simulink library "RspLib"  (R2018b)
settings: Solver=VariableStepAuto  StartTime=0.0  StopTime=10.0  RelTol=1e-3
undefined symbols (not defined in the file or in its folder): HMIRsp1, PassRsp1, RclRspStat1
libraries: $bdroot x22
settings Model: Creator=sn2xws  LastModifiedBy=sn2xws

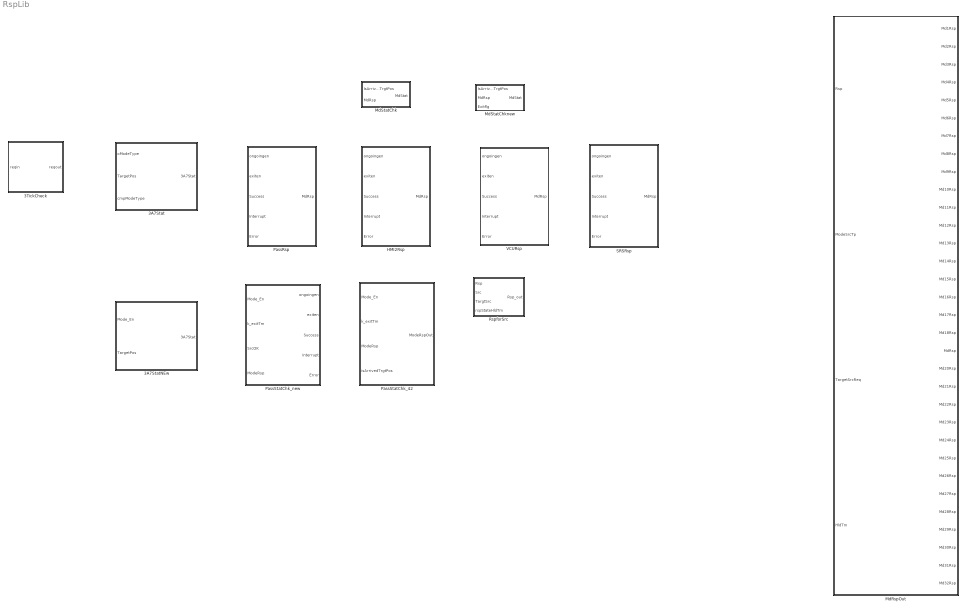
== system RspLib ==
  3A7Stat : Subsystem
  3A7StatNEw : Subsystem
  3TickCheck : Subsystem
  HMI2Rsp : Subsystem
  MdRspOut : Subsystem
  MdStatChk : Subsystem
  MdStatChknew : Subsystem
  PassRsp : Subsystem
  PassStatChk_42 : Stateflow chart  TreatAsAtomicUnit=on
  PassStatChk_new : Stateflow chart  TreatAsAtomicUnit=on
  RspforSrc : Subsystem
  SRSRsp : Subsystem
  VCURsp : Subsystem

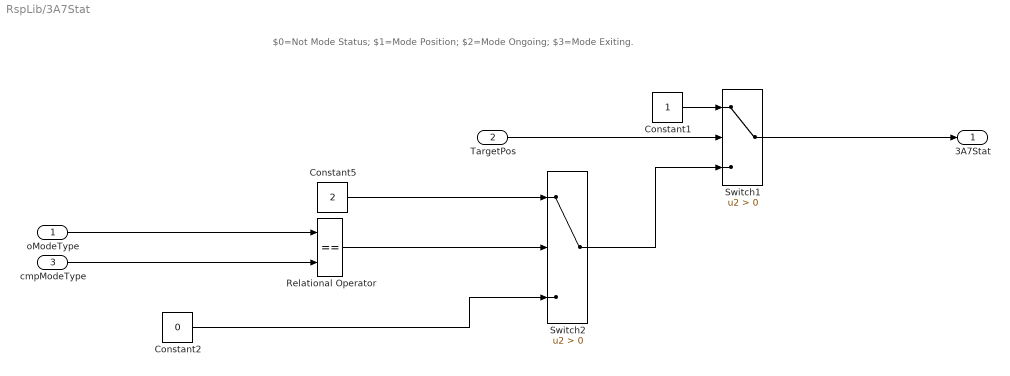
== system RspLib/3A7Stat ==
  note: $0=Not Mode Status; $1=Mode Position; $2=Mode Ongoing; $3=Mode Exiting.
  oModeType : Inport
  TargetPos : Inport  Port=2
  cmpModeType : Inport  Port=3
  Constant1 : Constant  OutDataTypeStr=uint8
  Constant2 : Constant  Value=0  OutDataTypeStr=uint8
  Constant5 : Constant  Value=2  OutDataTypeStr=uint8
  Relational Operator : RelationalOperator  Operator===  OutDataTypeStr=boolean  RndMeth=Simplest
  Switch1 : Switch  Criteria=u2 > Threshold
  Switch2 : Switch  Criteria=u2 > Threshold
  3A7Stat : Outport
  wires:
  Constant5/1 -> Switch2/1
  cmpModeType/1 -> Relational Operator/2
  TargetPos/1 -> Switch1/2
  Constant1/1 -> Switch1/1
  Relational Operator/1 -> Switch2/2
  oModeType/1 -> Relational Operator/1
  Switch1/1 -> 3A7Stat/1
  Constant2/1 -> Switch2/3
  Switch2/1 -> Switch1/3

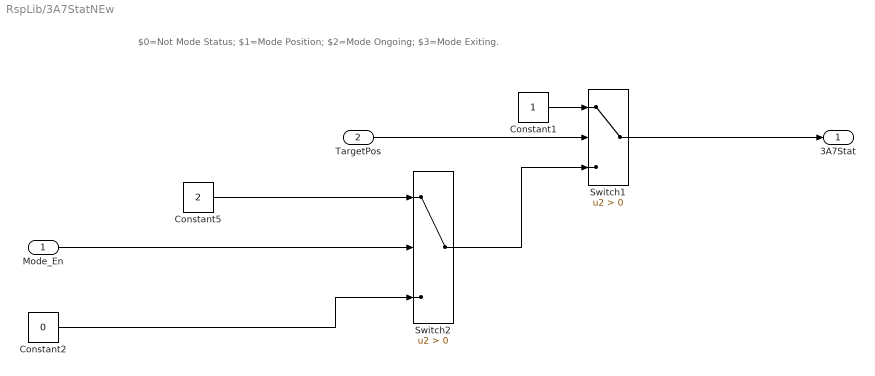
== system RspLib/3A7StatNEw ==
  note: $0=Not Mode Status; $1=Mode Position; $2=Mode Ongoing; $3=Mode Exiting.
  Mode_En : Inport
  TargetPos : Inport  Port=2
  Constant1 : Constant  OutDataTypeStr=uint8
  Constant2 : Constant  Value=0  OutDataTypeStr=uint8
  Constant5 : Constant  Value=2  OutDataTypeStr=uint8
  Switch1 : Switch  Criteria=u2 > Threshold
  Switch2 : Switch  Criteria=u2 > Threshold
  3A7Stat : Outport
  wires:
  Switch2/1 -> Switch1/3
  Constant2/1 -> Switch2/3
  Switch1/1 -> 3A7Stat/1
  Constant1/1 -> Switch1/1
  TargetPos/1 -> Switch1/2
  Constant5/1 -> Switch2/1
  Mode_En/1 -> Switch2/2

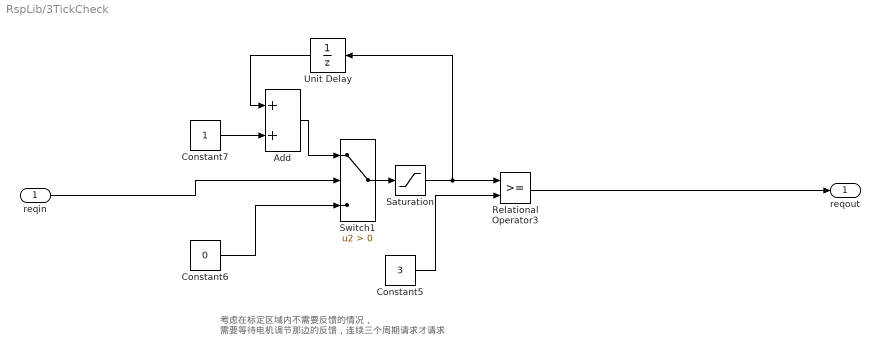
== system RspLib/3TickCheck ==
  note: 考虑在标定区域内不需要反馈的情况，
      | 需要等待电机调节那边的反馈，连续三个周期请求才请求
  reqin : Inport
  Add : Sum
  Constant5 : Constant  Value=3  OutDataTypeStr=uint8
  Constant6 : Constant  Value=0  OutDataTypeStr=uint8
  Constant7 : Constant  OutDataTypeStr=uint8
  Relational Operator3 : RelationalOperator  OutDataTypeStr=boolean  RndMeth=Simplest
  Saturation : Saturate  UpperLimit=3  LowerLimit=0  OutDataTypeStr=uint8
  Switch1 : Switch  Criteria=u2 > Threshold
  Unit Delay : UnitDelay  SampleTime=-1
  reqout : Outport
  wires:
  Unit Delay/1 -> Add/1
  Constant6/1 -> Switch1/3
  Constant5/1 -> Relational Operator3/2
  Constant7/1 -> Add/2
  Saturation/1 -> Unit Delay/1, Relational Operator3/1
  Add/1 -> Switch1/1
  Switch1/1 -> Saturation/1
  reqin/1 -> Switch1/2
  Relational Operator3/1 -> reqout/1

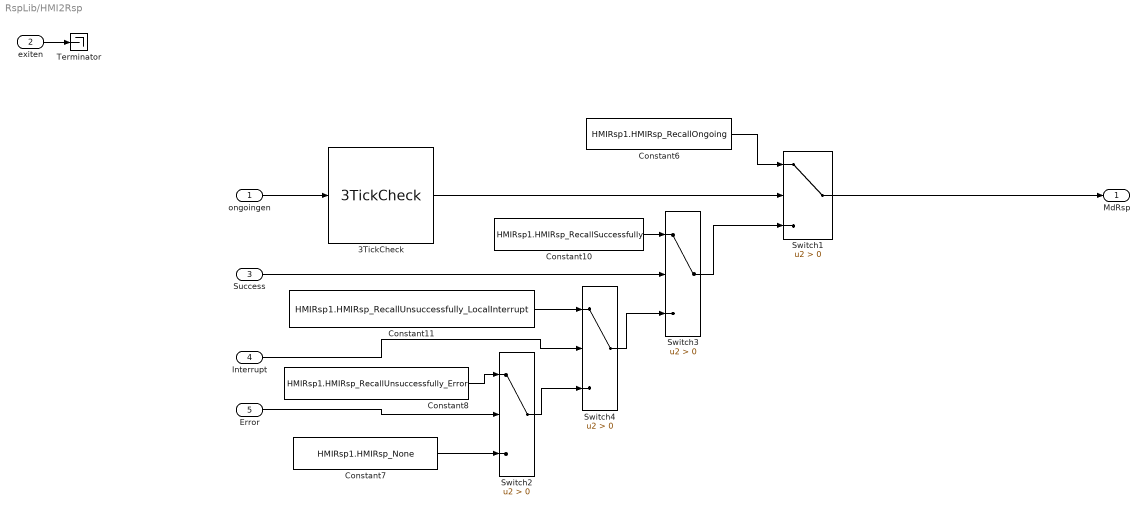
== system RspLib/HMI2Rsp ==
  ongoingen : Inport
  exiten : Inport  Port=2
  Success : Inport  Port=3
  Interrupt : Inport  Port=4
  Error : Inport  Port=5
  3TickCheck : $bdroot/3TickCheck  SystemSampleTime=-1
  Constant10 : Constant  Value=HMIRsp1.HMIRsp_RecallSuccessfully  OutDataTypeStr=Enum:HMIRsp1  SampleTime=-1
  Constant11 : Constant  Value=HMIRsp1.HMIRsp_RecallUnsuccessfully_LocalInterrupt  OutDataTypeStr=Enum:HMIRsp1  SampleTime=-1
  Constant6 : Constant  Value=HMIRsp1.HMIRsp_RecallOngoing  OutDataTypeStr=Enum:HMIRsp1  SampleTime=-1
  Constant7 : Constant  Value=HMIRsp1.HMIRsp_None  OutDataTypeStr=Enum:HMIRsp1  SampleTime=-1
  Constant8 : Constant  Value=HMIRsp1.HMIRsp_RecallUnsuccessfully_Error  OutDataTypeStr=Enum:HMIRsp1  SampleTime=-1
  Switch{1..4} (4 alike) : Switch  Criteria=u2 > Threshold
  Terminator : Terminator
  MdRsp : Outport  VectorParamsAs1DForOutWhenUnconnected=on
  wires:
  Constant10/1 -> Switch3/1
  Switch3/1 -> Switch1/3
  Switch1/1 -> MdRsp/1
  Constant6/1 -> Switch1/1
  Success/1 -> Switch3/2
  Switch2/1 -> Switch4/3
  Constant8/1 -> Switch2/1
  Constant11/1 -> Switch4/1
  Constant7/1 -> Switch2/3
  Switch4/1 -> Switch3/3
  ongoingen/1 -> 3TickCheck/1
  Interrupt/1 -> Switch4/2
  Error/1 -> Switch2/2
  exiten/1 -> Terminator/1
  3TickCheck/1 -> Switch1/2

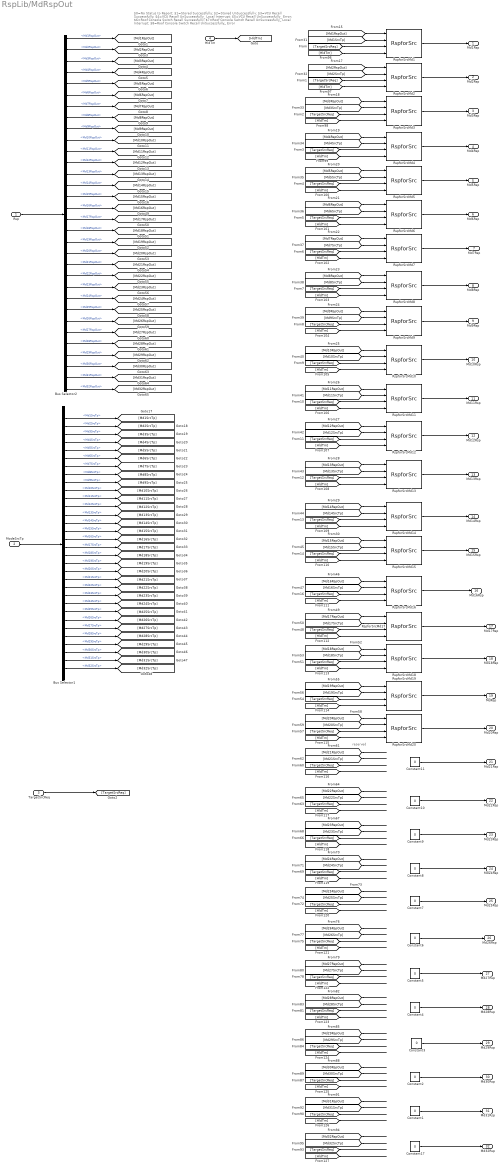
== system RspLib/MdRspOut ==
  note: $0=No Status to Report; $1=Stored Successfully; $2=Stored UnSuccessfully; $3=VCU Recall Successfully; $4=VCU Recall UnSuccessfully_ Local Interrupt; $5=VCU Recall UnSuccessfully_ Error; $6=Roof Console Switch Recall Successfully; $7=Roof Console Switch Recall UnSuccessfully_ Local Interrupt; $8=Roof Console Switch Recall UnSuccessfully_ Error
  note: reserved
  Rsp : Inport
  ModeSrcTp : Inport  Port=2
  TargetSrcReq : Inport  Port=3
  HldTm : Inport  Port=4
  Bus Selector1 : BusSelector  OutputSignals=Md1SrcTp,Md2SrcTp,Md3SrcTp,Md4SrcTp,Md5SrcTp,Md6SrcTp,Md7SrcTp,Md8SrcTp,Md9SrcTp,Md10SrcTp,Md11SrcTp,Md12SrcTp,Md13SrcTp,Md14SrcTp,Md15SrcTp,Md16SrcTp,Md17SrcTp,Md18SrcTp,Md19SrcTp,Md20SrcTp,Md21SrcTp,Md22SrcTp,Md23SrcTp,Md24SrcTp,Md25SrcTp,Md26SrcTp,Md27SrcTp,Md28SrcTp,Md29SrcTp,Md30SrcTp,Md31SrcTp,Md32SrcTp
  Bus Selector2 : BusSelector  OutputSignals=Md1RspOut,Md2RspOut,Md3RspOut,Md4RspOut,Md5RspOut,Md6RspOut,Md7RspOut,Md8RspOut,Md9RspOut,Md10RspOut,Md11RspOut,Md12RspOut,Md13RspOut,Md14RspOut,Md15RspOut,Md16RspOut,Md17RspOut,Md18RspOut,Md19RspOut,Md20RspOut,Md21RspOut,Md22RspOut,Md23RspOut,Md24RspOut,Md25RspOut,Md26RspOut,Md27RspOut,Md28RspOut,Md29RspOut,Md30RspOut,Md31RspOut,Md32RspOut
  Constant{1..11,17} (12 alike) : Constant  Value=0  OutDataTypeStr=uint8
  RspforSrcMd{1..20} (20 alike) : $bdroot/RspforSrc  SystemSampleTime=-1
  Md1Rsp : Outport  VectorParamsAs1DForOutWhenUnconnected=on
  Md2Rsp : Outport  Port=2  VectorParamsAs1DForOutWhenUnconnected=on
  Md3Rsp : Outport  Port=3  VectorParamsAs1DForOutWhenUnconnected=on
  Md4Rsp : Outport  Port=4  VectorParamsAs1DForOutWhenUnconnected=on
  Md5Rsp : Outport  Port=5  VectorParamsAs1DForOutWhenUnconnected=on
  Md6Rsp : Outport  Port=6  VectorParamsAs1DForOutWhenUnconnected=on
  Md7Rsp : Outport  Port=7  VectorParamsAs1DForOutWhenUnconnected=on
  Md8Rsp : Outport  Port=8  VectorParamsAs1DForOutWhenUnconnected=on
  Md9Rsp : Outport  Port=9  VectorParamsAs1DForOutWhenUnconnected=on
  Md10Rsp : Outport  Port=10  VectorParamsAs1DForOutWhenUnconnected=on
  Md11Rsp : Outport  Port=11  VectorParamsAs1DForOutWhenUnconnected=on
  Md12Rsp : Outport  Port=12  VectorParamsAs1DForOutWhenUnconnected=on
  Md13Rsp : Outport  Port=13  VectorParamsAs1DForOutWhenUnconnected=on
  Md14Rsp : Outport  Port=14  VectorParamsAs1DForOutWhenUnconnected=on
  Md15Rsp : Outport  Port=15  VectorParamsAs1DForOutWhenUnconnected=on
  Md16Rsp : Outport  Port=16  VectorParamsAs1DForOutWhenUnconnected=on
  Md17Rsp : Outport  Port=17  VectorParamsAs1DForOutWhenUnconnected=on
  Md18Rsp : Outport  Port=18  VectorParamsAs1DForOutWhenUnconnected=on
  MdRsp : Outport  Port=19  VectorParamsAs1DForOutWhenUnconnected=on
  Md20Rsp : Outport  Port=20  VectorParamsAs1DForOutWhenUnconnected=on
  Md21Rsp : Outport  Port=21  VectorParamsAs1DForOutWhenUnconnected=on
  Md22Rsp : Outport  Port=22  VectorParamsAs1DForOutWhenUnconnected=on
  Md23Rsp : Outport  Port=23  VectorParamsAs1DForOutWhenUnconnected=on
  Md24Rsp : Outport  Port=24  VectorParamsAs1DForOutWhenUnconnected=on
  Md25Rsp : Outport  Port=25  VectorParamsAs1DForOutWhenUnconnected=on
  Md26Rsp : Outport  Port=26  VectorParamsAs1DForOutWhenUnconnected=on
  Md27Rsp : Outport  Port=27  VectorParamsAs1DForOutWhenUnconnected=on
  Md28Rsp : Outport  Port=28  VectorParamsAs1DForOutWhenUnconnected=on
  Md29Rsp : Outport  Port=29  VectorParamsAs1DForOutWhenUnconnected=on
  Md30Rsp : Outport  Port=30  VectorParamsAs1DForOutWhenUnconnected=on
  Md31Rsp : Outport  Port=31  VectorParamsAs1DForOutWhenUnconnected=on
  Md32Rsp : Outport  Port=32  VectorParamsAs1DForOutWhenUnconnected=on
  wires:
  [TargetSrcReq] -> ?
  [Md32RspOut] -> ?
  [Md32SrcTp] -> ?
  [Md31SrcTp] -> ?
  [Md31RspOut] -> ?
  [TargetSrcReq] -> ?
  [TargetSrcReq] -> ?
  [Md30RspOut] -> ?
  [Md30SrcTp] -> ?
  [Md29SrcTp] -> ?
  [Md29RspOut] -> ?
  [TargetSrcReq] -> ?
  [TargetSrcReq] -> ?
  [Md28RspOut] -> ?
  [Md28SrcTp] -> ?
  [Md27SrcTp] -> ?
  [Md27RspOut] -> ?
  [TargetSrcReq] -> ?
  [TargetSrcReq] -> ?
  [Md26RspOut] -> ?
  [Md26SrcTp] -> ?
  [Md25SrcTp] -> ?
  [Md25RspOut] -> ?
  [TargetSrcReq] -> ?
  [TargetSrcReq] -> ?
  [Md24RspOut] -> ?
  [Md24SrcTp] -> ?
  [Md23SrcTp] -> ?
  [Md23RspOut] -> ?
  [TargetSrcReq] -> ?
  [TargetSrcReq] -> ?
  [Md22RspOut] -> ?
  [Md22SrcTp] -> ?
  [Md21SrcTp] -> ?
  [Md21RspOut] -> ?
  [TargetSrcReq] -> ?
  [TargetSrcReq] -> RspforSrcMd20/3
  [Md20RspOut] -> RspforSrcMd20/1
  [Md20SrcTp] -> RspforSrcMd20/2
  [Md19SrcTp] -> RspforSrcMd19/2
  [Md19RspOut] -> RspforSrcMd19/1
  [TargetSrcReq] -> RspforSrcMd19/3
  [TargetSrcReq] -> RspforSrcMd18/3
  [Md18RspOut] -> RspforSrcMd18/1
  [Md18SrcTp] -> RspforSrcMd18/2
  Bus Selector2/32 -> [Md32RspOut]  "<Md32RspOut>"
  Bus Selector2/31 -> [Md31RspOut]  "<Md31RspOut>"
  Bus Selector2/30 -> [Md30RspOut]  "<Md30RspOut>"
  Bus Selector2/29 -> [Md29RspOut]  "<Md29RspOut>"
  Bus Selector2/28 -> [Md28RspOut]  "<Md28RspOut>"
  Bus Selector2/27 -> [Md27RspOut]  "<Md27RspOut>"
  Bus Selector2/26 -> [Md26RspOut]  "<Md26RspOut>"
  Bus Selector2/25 -> [Md25RspOut]  "<Md25RspOut>"
  Bus Selector2/24 -> [Md24RspOut]  "<Md24RspOut>"
  Bus Selector2/23 -> [Md23RspOut]  "<Md23RspOut>"
  Bus Selector2/22 -> [Md22RspOut]  "<Md22RspOut>"
  Bus Selector2/21 -> [Md21RspOut]  "<Md21RspOut>"
  Bus Selector2/20 -> [Md20RspOut]  "<Md20RspOut>"
  Bus Selector2/19 -> [Md19RspOut]  "<Md19RspOut>"
  Bus Selector2/18 -> [Md18RspOut]  "<Md18RspOut>"
  Bus Selector2/17 -> [Md17RspOut]  "<Md17RspOut>"
  Bus Selector2/16 -> [Md16RspOut]  "<Md16RspOut>"
  [Md17SrcTp] -> RspforSrcMd17/2
  [Md17RspOut] -> RspforSrcMd17/1
  [TargetSrcReq] -> RspforSrcMd17/3
  [TargetSrcReq] -> RspforSrcMd16/3
  [Md16RspOut] -> RspforSrcMd16/1
  [Md16SrcTp] -> RspforSrcMd16/2
  Bus Selector1/32 -> [Md32SrcTp]  "<Md32SrcTp>"
  Bus Selector1/31 -> [Md31SrcTp]  "<Md31SrcTp>"
  Bus Selector1/30 -> [Md30SrcTp]  "<Md30SrcTp>"
  Bus Selector1/29 -> [Md29SrcTp]  "<Md29SrcTp>"
  Bus Selector1/28 -> [Md28SrcTp]  "<Md28SrcTp>"
  Bus Selector1/27 -> [Md27SrcTp]  "<Md27SrcTp>"
  Bus Selector1/26 -> [Md26SrcTp]  "<Md26SrcTp>"
  Bus Selector1/25 -> [Md25SrcTp]  "<Md25SrcTp>"
  Bus Selector1/24 -> [Md24SrcTp]  "<Md24SrcTp>"
  Bus Selector1/23 -> [Md23SrcTp]  "<Md23SrcTp>"
  Bus Selector1/22 -> [Md22SrcTp]  "<Md22SrcTp>"
  Bus Selector1/21 -> [Md21SrcTp]  "<Md21SrcTp>"
  Bus Selector1/20 -> [Md20SrcTp]  "<Md20SrcTp>"
  Bus Selector1/19 -> [Md19SrcTp]  "<Md19SrcTp>"
  Bus Selector1/18 -> [Md18SrcTp]  "<Md18SrcTp>"
  Bus Selector1/17 -> [Md17SrcTp]  "<Md17SrcTp>"
  Bus Selector1/16 -> [Md16SrcTp]  "<Md16SrcTp>"
  [Md14SrcTp] -> RspforSrcMd14/2
  [Md13SrcTp] -> RspforSrcMd13/2
  [Md15SrcTp] -> RspforSrcMd15/2
  [Md12SrcTp] -> RspforSrcMd12/2
  [Md11SrcTp] -> RspforSrcMd11/2
  [Md10SrcTp] -> RspforSrcMd10/2
  [Md9SrcTp] -> RspforSrcMd9/2
  [Md8SrcTp] -> RspforSrcMd8/2
  [Md7SrcTp] -> RspforSrcMd7/2
  [Md6SrcTp] -> RspforSrcMd6/2
  [Md5SrcTp] -> RspforSrcMd5/2
  [Md4SrcTp] -> RspforSrcMd4/2
  [Md3SrcTp] -> RspforSrcMd3/2
  [Md2SrcTp] -> RspforSrcMd2/2
  Bus Selector1/15 -> [Md15SrcTp]  "<Md15SrcTp>"
  Bus Selector1/14 -> [Md14SrcTp]  "<Md14SrcTp>"
  Bus Selector1/13 -> [Md13SrcTp]  "<Md13SrcTp>"
  Bus Selector1/12 -> [Md12SrcTp]  "<Md12SrcTp>"
  Bus Selector1/11 -> [Md11SrcTp]  "<Md11SrcTp>"
  Bus Selector1/10 -> [Md10SrcTp]  "<Md10SrcTp>"
  Bus Selector1/9 -> [Md9SrcTp]  "<Md9SrcTp>"
  Bus Selector1/8 -> [Md8SrcTp]  "<Md8SrcTp>"
  Bus Selector1/7 -> [Md7SrcTp]  "<Md7SrcTp>"
  Bus Selector1/6 -> [Md6SrcTp]  "<Md6SrcTp>"
  Bus Selector1/5 -> [Md5SrcTp]  "<Md5SrcTp>"
  Bus Selector1/4 -> [Md4SrcTp]  "<Md4SrcTp>"
  Bus Selector1/3 -> [Md3SrcTp]  "<Md3SrcTp>"
  Bus Selector1/2 -> [Md2SrcTp]  "<Md2SrcTp>"
  Bus Selector1/1 -> [Md1SrcTp]  "<Md1SrcTp>"
  Constant7/1 -> Md25Rsp/1
  [Md15RspOut] -> RspforSrcMd15/1
  [Md14RspOut] -> RspforSrcMd14/1
  [Md13RspOut] -> RspforSrcMd13/1
  [Md12RspOut] -> RspforSrcMd12/1
  [Md11RspOut] -> RspforSrcMd11/1
  [Md10RspOut] -> RspforSrcMd10/1
  [Md9RspOut] -> RspforSrcMd9/1
  [Md8RspOut] -> RspforSrcMd8/1
  [Md7RspOut] -> RspforSrcMd7/1
  [Md6RspOut] -> RspforSrcMd6/1
  [Md5RspOut] -> RspforSrcMd5/1
  [Md4RspOut] -> RspforSrcMd4/1
  [Md3RspOut] -> RspforSrcMd3/1
  [Md2RspOut] -> RspforSrcMd2/1
  RspforSrcMd15/1 -> Md15Rsp/1
  RspforSrcMd14/1 -> Md14Rsp/1
  RspforSrcMd13/1 -> Md13Rsp/1
  RspforSrcMd12/1 -> Md12Rsp/1
  RspforSrcMd11/1 -> Md11Rsp/1
  RspforSrcMd10/1 -> Md10Rsp/1
  RspforSrcMd9/1 -> Md9Rsp/1
  RspforSrcMd8/1 -> Md8Rsp/1
  RspforSrcMd7/1 -> Md7Rsp/1
  RspforSrcMd6/1 -> Md6Rsp/1
  RspforSrcMd5/1 -> Md5Rsp/1
  RspforSrcMd4/1 -> Md4Rsp/1
  RspforSrcMd3/1 -> Md3Rsp/1
  RspforSrcMd2/1 -> Md2Rsp/1
  RspforSrcMd1/1 -> Md1Rsp/1
  [TargetSrcReq] -> RspforSrcMd1/3
  [Md1SrcTp] -> RspforSrcMd1/2
  [Md1RspOut] -> RspforSrcMd1/1
  [TargetSrcReq] -> RspforSrcMd15/3
  [TargetSrcReq] -> RspforSrcMd14/3
  [TargetSrcReq] -> RspforSrcMd13/3
  [TargetSrcReq] -> RspforSrcMd12/3
  [TargetSrcReq] -> RspforSrcMd11/3
  RspforSrcMd17/1 -> Md17Rsp/1
  RspforSrcMd18/1 -> Md18Rsp/1
  RspforSrcMd19/1 -> MdRsp/1
  RspforSrcMd20/1 -> Md20Rsp/1
  Constant11/1 -> Md21Rsp/1
  Constant10/1 -> Md22Rsp/1
  Constant9/1 -> Md23Rsp/1
  Constant8/1 -> Md24Rsp/1
  Constant6/1 -> Md26Rsp/1
  [TargetSrcReq] -> RspforSrcMd10/3
  [TargetSrcReq] -> RspforSrcMd9/3
  [TargetSrcReq] -> RspforSrcMd8/3
  [TargetSrcReq] -> RspforSrcMd7/3
  [TargetSrcReq] -> RspforSrcMd6/3
  [TargetSrcReq] -> RspforSrcMd5/3
  [TargetSrcReq] -> RspforSrcMd4/3
  [TargetSrcReq] -> RspforSrcMd3/3
  [TargetSrcReq] -> RspforSrcMd2/3
  Bus Selector2/15 -> [Md15RspOut]  "<Md15RspOut>"
  Bus Selector2/14 -> [Md14RspOut]  "<Md14RspOut>"
  Bus Selector2/13 -> [Md13RspOut]  "<Md13RspOut>"
  Bus Selector2/12 -> [Md12RspOut]  "<Md12RspOut>"
  Bus Selector2/11 -> [Md11RspOut]  "<Md11RspOut>"
  Bus Selector2/10 -> [Md10RspOut]  "<Md10RspOut>"
  Bus Selector2/9 -> [Md9RspOut]  "<Md9RspOut>"
  Bus Selector2/8 -> [Md8RspOut]  "<Md8RspOut>"
  Bus Selector2/7 -> [Md7RspOut]  "<Md7RspOut>"
  Bus Selector2/6 -> [Md6RspOut]  "<Md6RspOut>"
  Bus Selector2/5 -> [Md5RspOut]  "<Md5RspOut>"
  Bus Selector2/4 -> [Md4RspOut]  "<Md4RspOut>"
  Bus Selector2/3 -> [Md3RspOut]  "<Md3RspOut>"
  Bus Selector2/2 -> [Md2RspOut]  "<Md2RspOut>"
  Bus Selector2/1 -> [Md1RspOut]  "<Md1RspOut>"
  TargetSrcReq/1 -> [TargetSrcReq]
  ModeSrcTp/1 -> Bus Selector1/1
  Constant5/1 -> Md27Rsp/1
  Constant4/1 -> Md28Rsp/1
  Constant3/1 -> Md29Rsp/1
  Constant2/1 -> Md30Rsp/1
  Constant1/1 -> Md31Rsp/1
  Constant17/1 -> Md32Rsp/1
  Rsp/1 -> Bus Selector2/1
  [HldTm] -> RspforSrcMd1/4
  [HldTm] -> RspforSrcMd2/4
  [HldTm] -> RspforSrcMd3/4
  [HldTm] -> RspforSrcMd4/4
  [HldTm] -> RspforSrcMd5/4
  [HldTm] -> RspforSrcMd6/4
  [HldTm] -> RspforSrcMd7/4
  [HldTm] -> RspforSrcMd8/4
  [HldTm] -> RspforSrcMd9/4
  [HldTm] -> RspforSrcMd10/4
  [HldTm] -> RspforSrcMd11/4
  [HldTm] -> RspforSrcMd12/4
  [HldTm] -> RspforSrcMd13/4
  [HldTm] -> RspforSrcMd14/4
  [HldTm] -> RspforSrcMd15/4
  [HldTm] -> RspforSrcMd16/4
  [HldTm] -> RspforSrcMd17/4
  [HldTm] -> RspforSrcMd18/4
  [HldTm] -> RspforSrcMd19/4
  [HldTm] -> RspforSrcMd20/4
  [HldTm] -> ?
  [HldTm] -> ?
  [HldTm] -> ?
  [HldTm] -> ?
  [HldTm] -> ?
  [HldTm] -> ?
  [HldTm] -> ?
  [HldTm] -> ?
  [HldTm] -> ?
  [HldTm] -> ?
  [HldTm] -> ?
  [HldTm] -> ?
  HldTm/1 -> [HldTm]
  RspforSrcMd16/1 -> Md16Rsp/1

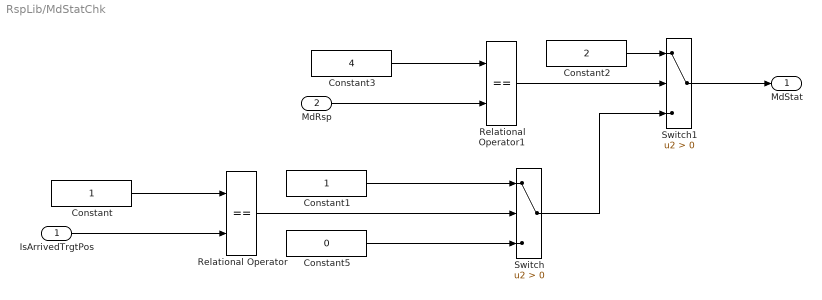
== system RspLib/MdStatChk ==
  IsArrivedTrgtPos : Inport
  MdRsp : Inport  Port=2
  Constant : Constant  OutDataTypeStr=boolean
  Constant1 : Constant  OutDataTypeStr=uint8
  Constant2 : Constant  Value=2  OutDataTypeStr=uint8
  Constant3 : Constant  Value=4  OutDataTypeStr=uint8
  Constant5 : Constant  Value=0  OutDataTypeStr=uint8
  Relational Operator : RelationalOperator  Operator===  OutDataTypeStr=boolean  RndMeth=Simplest
  Relational Operator1 : RelationalOperator  Operator===  OutDataTypeStr=boolean  RndMeth=Simplest
  Switch : Switch  Criteria=u2 > Threshold
  Switch1 : Switch  Criteria=u2 > Threshold
  MdStat : Outport
  wires:
  Constant3/1 -> Relational Operator1/1
  MdRsp/1 -> Relational Operator1/2
  Constant2/1 -> Switch1/1
  Relational Operator1/1 -> Switch1/2
  Constant1/1 -> Switch/1
  Constant/1 -> Relational Operator/1
  IsArrivedTrgtPos/1 -> Relational Operator/2
  Relational Operator/1 -> Switch/2
  Constant5/1 -> Switch/3
  Switch/1 -> Switch1/3
  Switch1/1 -> MdStat/1

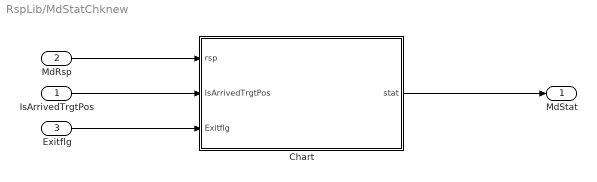
== system RspLib/MdStatChknew ==
  IsArrivedTrgtPos : Inport
  MdRsp : Inport  Port=2
  Exitflg : Inport  Port=3
  Chart : Stateflow chart  TreatAsAtomicUnit=on
  MdStat : Outport
  wires:
  MdRsp/1 -> Chart/1(rsp)
  Exitflg/1 -> Chart/3(Exitflg)
  IsArrivedTrgtPos/1 -> Chart/2(IsArrivedTrgtPos)
  Chart/1(stat) -> MdStat/1

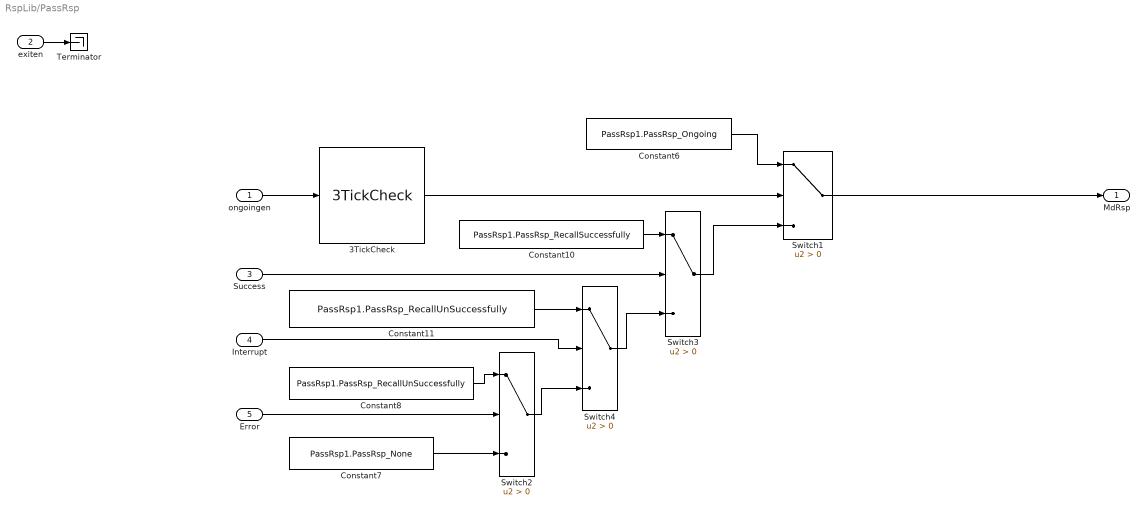
== system RspLib/PassRsp ==
  ongoingen : Inport
  exiten : Inport  Port=2
  Success : Inport  Port=3
  Interrupt : Inport  Port=4
  Error : Inport  Port=5
  3TickCheck : $bdroot/3TickCheck  SystemSampleTime=-1
  Constant10 : Constant  Value=PassRsp1.PassRsp_RecallSuccessfully  OutDataTypeStr=Enum:PassRsp1  SampleTime=-1
  Constant11 : Constant  Value=PassRsp1.PassRsp_RecallUnSuccessfully  OutDataTypeStr=Enum:PassRsp1  SampleTime=-1
  Constant6 : Constant  Value=PassRsp1.PassRsp_Ongoing  OutDataTypeStr=Enum:PassRsp1  SampleTime=-1
  Constant7 : Constant  Value=PassRsp1.PassRsp_None  OutDataTypeStr=Enum:PassRsp1  SampleTime=-1
  Constant8 : Constant  Value=PassRsp1.PassRsp_RecallUnSuccessfully  OutDataTypeStr=Enum:PassRsp1  SampleTime=-1
  Switch{1..4} (4 alike) : Switch  Criteria=u2 > Threshold
  Terminator : Terminator
  MdRsp : Outport  VectorParamsAs1DForOutWhenUnconnected=on
  wires:
  exiten/1 -> Terminator/1
  Error/1 -> Switch2/2
  Interrupt/1 -> Switch4/2
  ongoingen/1 -> 3TickCheck/1
  Switch4/1 -> Switch3/3
  Constant7/1 -> Switch2/3
  Constant11/1 -> Switch4/1
  Constant8/1 -> Switch2/1
  Switch2/1 -> Switch4/3
  Success/1 -> Switch3/2
  Constant6/1 -> Switch1/1
  Switch1/1 -> MdRsp/1
  Switch3/1 -> Switch1/3
  Constant10/1 -> Switch3/1
  3TickCheck/1 -> Switch1/2

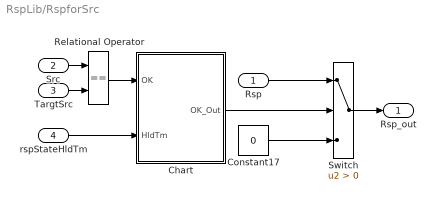
== system RspLib/RspforSrc ==
  Rsp : Inport
  Src : Inport  Port=2
  TargtSrc : Inport  Port=3
  rspStateHldTm : Inport  Port=4
  Chart : Stateflow chart  TreatAsAtomicUnit=on
  Constant17 : Constant  Value=0  OutDataTypeStr=uint8
  Relational Operator : RelationalOperator  Operator===  OutDataTypeStr=boolean  RndMeth=Simplest
  Switch : Switch  Criteria=u2 > Threshold
  Rsp_out : Outport
  wires:
  TargtSrc/1 -> Relational Operator/2
  Src/1 -> Relational Operator/1
  Switch/1 -> Rsp_out/1
  Constant17/1 -> Switch/3
  Rsp/1 -> Switch/1
  Chart/1(OK_Out) -> Switch/2
  Relational Operator/1 -> Chart/1(OK)
  rspStateHldTm/1 -> Chart/2(HldTm)

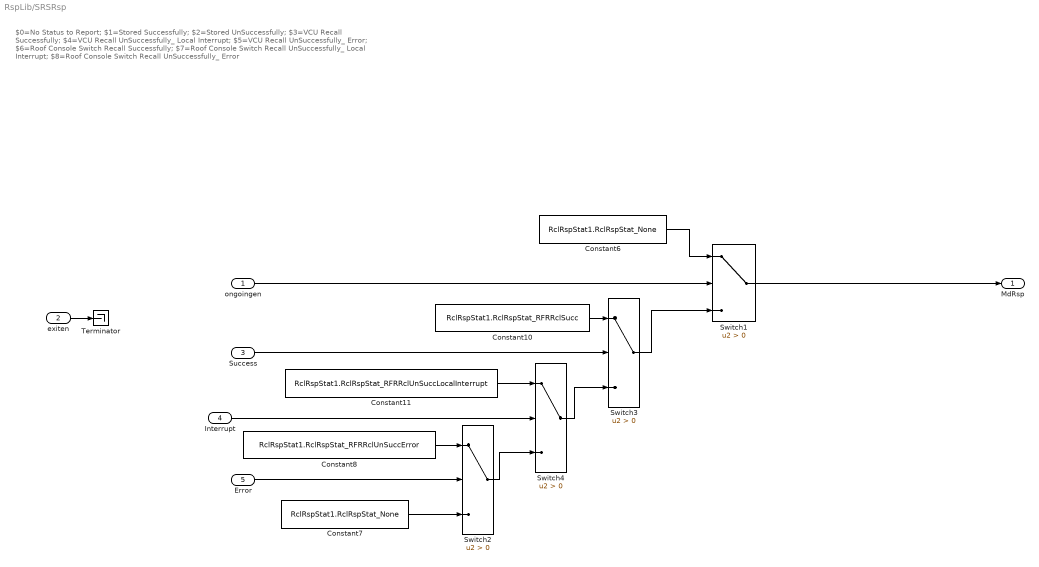
== system RspLib/SRSRsp ==
  note: $0=No Status to Report; $1=Stored Successfully; $2=Stored UnSuccessfully; $3=VCU Recall Successfully; $4=VCU Recall UnSuccessfully_ Local Interrupt; $5=VCU Recall UnSuccessfully_ Error; $6=Roof Console Switch Recall Successfully; $7=Roof Console Switch Recall UnSuccessfully_ Local Interrupt; $8=Roof Console Switch Recall UnSuccessfully_ Error
  ongoingen : Inport
  exiten : Inport  Port=2
  Success : Inport  Port=3
  Interrupt : Inport  Port=4
  Error : Inport  Port=5
  Constant10 : Constant  Value=RclRspStat1.RclRspStat_RFRRclSucc  OutDataTypeStr=Enum:RclRspStat1  SampleTime=-1
  Constant11 : Constant  Value=RclRspStat1.RclRspStat_RFRRclUnSuccLocalInterrupt  OutDataTypeStr=Enum:RclRspStat1  SampleTime=-1
  Constant6 : Constant  Value=RclRspStat1.RclRspStat_None  OutDataTypeStr=Enum:RclRspStat1  SampleTime=-1
  Constant7 : Constant  Value=RclRspStat1.RclRspStat_None  OutDataTypeStr=Enum:RclRspStat1  SampleTime=-1
  Constant8 : Constant  Value=RclRspStat1.RclRspStat_RFRRclUnSuccError  OutDataTypeStr=Enum:RclRspStat1  SampleTime=-1
  Switch{1..4} (4 alike) : Switch  Criteria=u2 > Threshold
  Terminator : Terminator
  MdRsp : Outport  VectorParamsAs1DForOutWhenUnconnected=on
  wires:
  exiten/1 -> Terminator/1
  Error/1 -> Switch2/2
  Interrupt/1 -> Switch4/2
  ongoingen/1 -> Switch1/2
  Switch4/1 -> Switch3/3
  Constant7/1 -> Switch2/3
  Constant11/1 -> Switch4/1
  Constant8/1 -> Switch2/1
  Switch2/1 -> Switch4/3
  Success/1 -> Switch3/2
  Constant6/1 -> Switch1/1
  Switch1/1 -> MdRsp/1
  Switch3/1 -> Switch1/3
  Constant10/1 -> Switch3/1

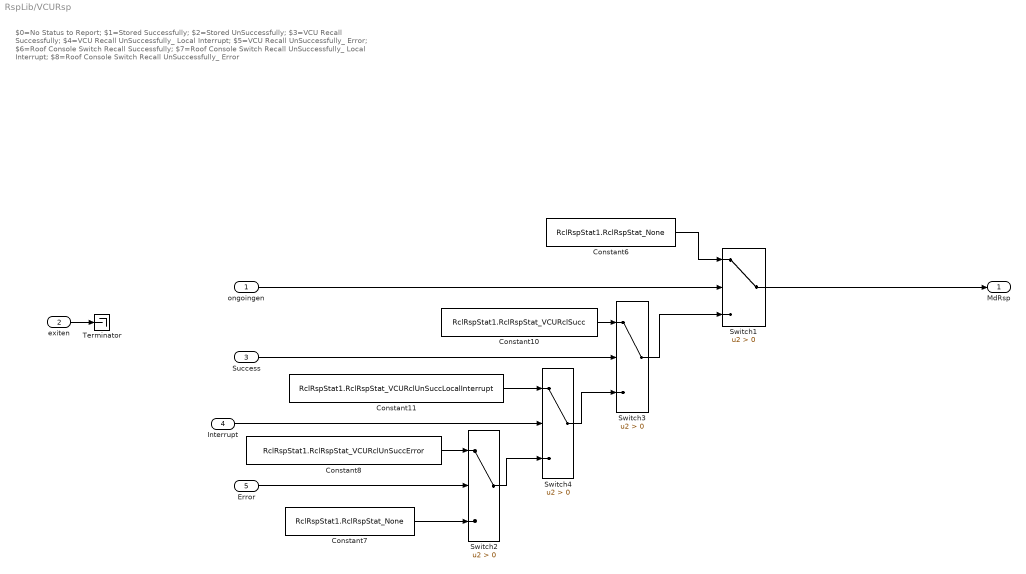
== system RspLib/VCURsp ==
  note: $0=No Status to Report; $1=Stored Successfully; $2=Stored UnSuccessfully; $3=VCU Recall Successfully; $4=VCU Recall UnSuccessfully_ Local Interrupt; $5=VCU Recall UnSuccessfully_ Error; $6=Roof Console Switch Recall Successfully; $7=Roof Console Switch Recall UnSuccessfully_ Local Interrupt; $8=Roof Console Switch Recall UnSuccessfully_ Error
  ongoingen : Inport
  exiten : Inport  Port=2
  Success : Inport  Port=3
  Interrupt : Inport  Port=4
  Error : Inport  Port=5
  Constant10 : Constant  Value=RclRspStat1.RclRspStat_VCURclSucc  OutDataTypeStr=Enum:RclRspStat1  SampleTime=-1
  Constant11 : Constant  Value=RclRspStat1.RclRspStat_VCURclUnSuccLocalInterrupt  OutDataTypeStr=Enum:RclRspStat1  SampleTime=-1
  Constant6 : Constant  Value=RclRspStat1.RclRspStat_None  OutDataTypeStr=Enum:RclRspStat1  SampleTime=-1
  Constant7 : Constant  Value=RclRspStat1.RclRspStat_None  OutDataTypeStr=Enum:RclRspStat1  SampleTime=-1
  Constant8 : Constant  Value=RclRspStat1.RclRspStat_VCURclUnSuccError  OutDataTypeStr=Enum:RclRspStat1  SampleTime=-1
  Switch{1..4} (4 alike) : Switch  Criteria=u2 > Threshold
  Terminator : Terminator
  MdRsp : Outport  VectorParamsAs1DForOutWhenUnconnected=on
  wires:
  Constant10/1 -> Switch3/1
  Switch3/1 -> Switch1/3
  Switch1/1 -> MdRsp/1
  Constant6/1 -> Switch1/1
  Success/1 -> Switch3/2
  Switch2/1 -> Switch4/3
  Constant8/1 -> Switch2/1
  Constant11/1 -> Switch4/1
  Constant7/1 -> Switch2/3
  Switch4/1 -> Switch3/3
  ongoingen/1 -> Switch1/2
  Interrupt/1 -> Switch4/2
  Error/1 -> Switch2/2
  exiten/1 -> Terminator/1

== stateflow chart RspLib/PassStatChk_new ==
  state othermode
    en:exiten=0;
    en:ongoingen = 0;
    en:cntexit = 1;
    en:Success = 0;
    en:Interrupt = 0;
    en:Error = 0;
  state cmpmode
    en:ongoingen=1;
    en:cntongoing = 0;
  state exitingsuccess
    en:ongoingen=0;
    en:exiten =1;
    en:Success = 1;
    du:cntexit++;
  state exitingInterrupt
    en:ongoingen=0;
    en:exiten =1;
    en:Interrupt =1;
    du:cntexit++;
  state exitingError
    en:ongoingen=0;
    en:exiten =1;
    en:Error =1;
    du:cntexit++;
  (default) -> othermode
  othermode -> cmpmode : [(Mode_En) &&SrcOK]
  exitingsuccess -> othermode : [cntexit>=k_exitTm]
  cmpmode -> exitingsuccess [order 1] : [(!Mode_En)&&...
      | (ModeRsp ==MdRsp_RecallSuccessfully)]
  exitingInterrupt -> othermode : [cntexit>=k_exitTm]
  cmpmode -> exitingInterrupt [order 2] : [(!Mode_En)&&...
      | (ModeRsp ==MdRsp_RecallUnsuccessfully_LocalInterrupt)]
  exitingError -> othermode : [cntexit>=k_exitTm]
  cmpmode -> exitingError [order 3] : [(!Mode_En)/*&&...
      | (ModeRsp ==MdRsp_RecallUnsuccessfully_Error)*/]
  data: ongoingen output boolean; exiten output boolean; Mode_En input boolean; k_exitTm input uint8; cntongoing local uint8; cntexit local uint8; SrcOK input boolean; ModeRsp input Enum: MdRspLocal1; Success output boolean; Interrupt output boolean; Error output boolean

== stateflow chart RspLib/PassStatChk_42 ==
  state othermode
    en:ModeRspOut =0;
    en:cntexit=1;
  state cmpmodeOngoing
    en:ModeRspOut =4;
  state TartPosAlready
    en:ModeRspOut =5;
    du:cntexit++;
  note: /*Change Request 147856
      | 在前提条件不满足、开关打断、防夹干涉导致模式中断时，
      | MSM需要先判断此模式是否已经满足调用成功的条件，
      | 若不满足，再报调用失败。210816*/
  state exitingsuccess
    en:ModeRspOut =1;
    du:cntexit++;
  state exitingInterrupt
    en:ModeRspOut =2;
    du:cntexit++;
  state exitingError
    en:ModeRspOut =3;
    du:cntexit++;
  (default) -> othermode
  othermode -> (junction 46) : [(Mode_En)]
  (junction 46) -> cmpmodeOngoing [order 2]
  (junction 46) -> TartPosAlready [order 1] : [isArrivedTrgtPos]
  TartPosAlready -> othermode : [cntexit>=k_exitTm]
  exitingsuccess -> othermode : [cntexit>=k_exitTm]
  cmpmodeOngoing -> exitingsuccess [order 1] : [(!Mode_En)&&...
      | (ModeRsp ==MdRsp_RecallSuccessfully||isArrivedTrgtPos)]
  exitingInterrupt -> othermode : [cntexit>=k_exitTm]
  cmpmodeOngoing -> exitingInterrupt [order 2] : [(!Mode_En)&&...
      | (ModeRsp ==MdRsp_RecallUnsuccessfully_LocalInterrupt)]
  exitingError -> othermode : [cntexit>=k_exitTm]
  cmpmodeOngoing -> exitingError [order 3] : [(!Mode_En)/*&&...
      | (ModeRsp ==MdRsp_RecallUnsuccessfully_Error)*/]
  data: Mode_En input boolean; k_exitTm input uint8; cntexit local uint8; ModeRsp input Enum: MdRspLocal1; ModeRspOut output uint8; isArrivedTrgtPos input boolean

== stateflow chart RspLib/RspforSrc/Chart ==
  state OK
    en:Cnt=0;
    en:OK_Out=1;
  state IDLE
    en:OK_Out=0;
  state WAIT
    en:Cnt=Cnt+1;
    du:Cnt=Cnt+1;
  (default) -> IDLE
  IDLE -> OK : [OK ==1]
  OK -> WAIT : [OK==0 ]
  WAIT -> IDLE [order 2] : [Cnt>=(HldTm)]
  WAIT -> OK [order 1] : [OK ==1]
  data: OK input boolean; HldTm input uint8; Cnt local uint8; OK_Out output boolean

== stateflow chart RspLib/MdStatChknew/Chart ==
  state idle
    en:stat = 0;
  state ongoing
    en:stat = 2;
  state ispos
    en:stat = 1;
  (default) -> idle
  idle -> ongoing [order 1] : [rsp==4]
  ongoing -> ispos [order 1] : [rsp==1]
  ongoing -> idle [order 2] : [rsp!=4]
  idle -> ispos [order 2] : [rsp==5]
  ispos -> idle : [!IsArrivedTrgtPos ||Exitflg]
  data: rsp input uint8; IsArrivedTrgtPos input boolean; Exitflg input boolean; stat output uint8
